simulink model "Identification_1degre"  (R2015a)
settings: Solver=ode3  StartTime=0.0  StopTime=10  FixedStep=0.01  RelTol=1e-3
InitFcn:
  | load('LeftOutput_Measures.mat');
  | load('LeftOutput_Measures.mat');
  | Parametres_Rover
undefined symbols (not defined in the file): KL, TdL, TL
settings Model: Creator=tbaroche  LastModifiedBy=tbaroche

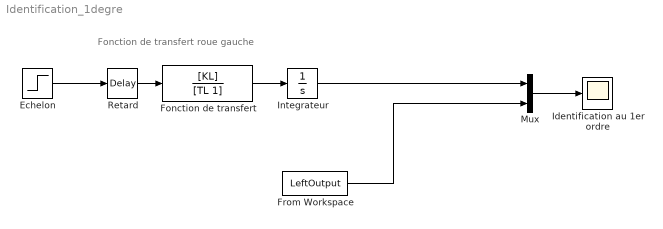
== system Identification_1degre ==
  note: Fonction de transfert roue gauche
  Echelon : Step  Time=3  After=50  SampleTime=0
  Fonction de transfert : TransferFcn  Numerator=[KL]  Denominator=[TL 1]
  From Workspace : FromWorkspace  VariableName=LeftOutput  SampleTime=0
  Identification au 1er ordre : Scope
      settings: YMin=-2000  YMax=12000
  Integrateur : Integrator
  Mux : Mux  Inputs=2
  Retard : TransportDelay  DelayTime=TdL
  wires:
  Mux/1 -> Identification au 1er ordre/1
  Integrateur/1 -> Mux/1
  From Workspace/1 -> Mux/2
  Retard/1 -> Fonction de transfert/1
  Fonction de transfert/1 -> Integrateur/1
  Echelon/1 -> Retard/1
